simulink model "three_sine_model"  (R2025b)
settings: Solver=VariableStepAuto  StartTime=0.0  StopTime=10.0  MaxStep=0.01  RelTol=1e-3

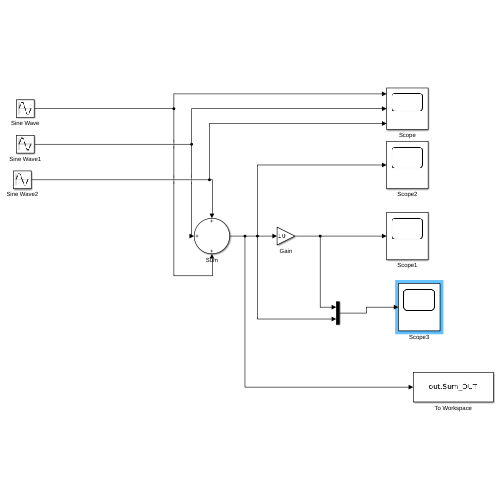
[thumbnail: Simulink's stored preview of the top-level diagram]
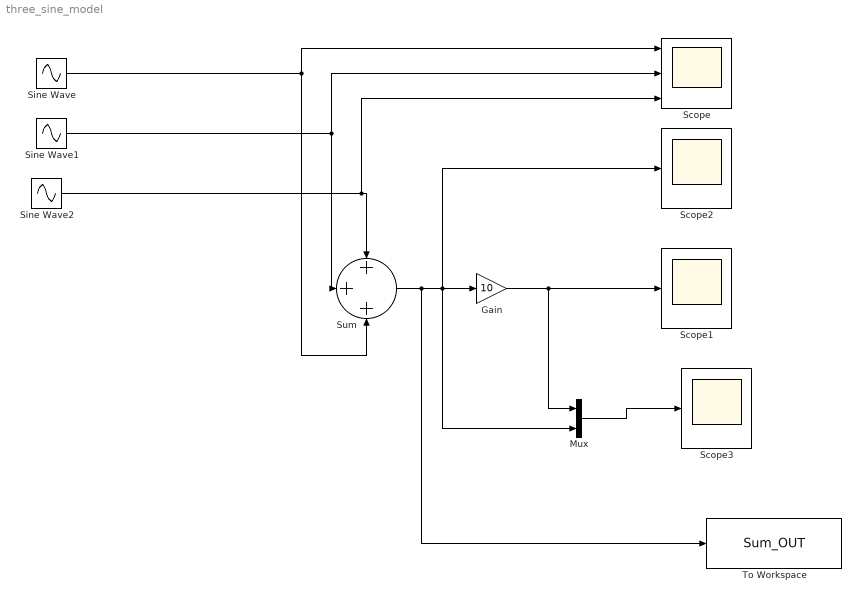
== system three_sine_model ==
  Gain : Gain  Gain=10
  Mux : Mux  Inputs=2
  Scope : Scope  NumInputPorts=3
      settings: ActiveDisplayYMinimum=-1.2499967500526621  ActiveDisplayYMaximum=1.2499992865967788
  Scope1 : Scope
      settings: ActiveDisplayYMinimum=-34.400175950066789  ActiveDisplayYMaximum=34.399800198065613
  Scope2 : Scope
      settings: ActiveDisplayYMinimum=-34.400175950066789  ActiveDisplayYMaximum=34.399800198065613  DataLoggingVariableName=ScopeData2
  Scope3 : Scope
      settings: ActiveDisplayYMinimum=-34.400175950066789  ActiveDisplayYMaximum=34.399800198065613  DataLoggingVariableName=ScopeData3
  Sine Wave : Sin  SampleTime=0
  Sine Wave1 : Sin  Frequency=5  SampleTime=0
  Sine Wave2 : Sin  Frequency=10  SampleTime=0
  Sum : Sum  Inputs=+++
  To Workspace : ToWorkspace  VariableName=Sum_OUT  SaveFormat=Timeseries  SampleTime=-1
  wires:
  Sine Wave/1 -> Sum/3, Scope/1
  Sine Wave1/1 -> Scope/2, Sum/2
  Sine Wave2/1 -> Scope/3, Sum/1
  Sum/1 -> To Workspace/1, Mux/2, Scope2/1, Gain/1
  Gain/1 -> Mux/1, Scope1/1
  Mux/1 -> Scope3/1
